simulink model "test_1_cs"  (R2020a)
settings: Solver=ode5  StartTime=0.0  StopTime=150  FixedStep=1/1000  RelTol=1e-3
PreLoadFcn:
  | mbxruntime.callbacks.PreLoadFcn(bdroot);
PostLoadFcn:
  | mbxruntime.callbacks.PostLoadFcn(bdroot);
InitFcn:
  | mbxruntime.callbacks.InitFcn(bdroot);
StartFcn:
  | mbxruntime.callbacks.StartFcn(bdroot);
StopFcn:
  | mbxruntime.callbacks.StopFcn(bdroot);
model workspace (MAT data in the model file):
  mbox_table : object (value not decoded)
  model_closed = 0
  sim_status = 0
undefined symbols (not defined in the file or in its folder): aubr, c_factor, cf, cr, DiscIntNeverNeededParam, global_path_x, global_path_y, KD_PID_distance, KD_PID_speed, KI_PID_distance, KI_PID_speed, KP_PID_distance, KP_PID_speed, la, lb, LQR_K1, LQR_K2, LQR_K3, LQR_K4, m, rack_displacement, right_wheel_ground, tablebr, vubr, vx_break_point
libraries: PreScanSimulinkLibrary x48, simulink_extras x5, simulink x3, Solver_SF x1
(part 8 of 12)

== system test_1_cs/Audi_A8_Sedan_1/control module/control main/longitudinal control double PID ==
  s_err[m] : Inport
  speed_desire[m/s] : Inport  Port=2
  accelerate desire[m/s^2] : Inport  Port=3
  host_speed[m/s] : Inport  Port=4
  host_s_dot[m/s] : Inport  Port=5
  KP_PID_distance : Inport  Port=6
  KI_PID_distance : Inport  Port=7
  KD_PID_distance : Inport  Port=8
  KP_PID_speed : Inport  Port=9
  KI_PID_speed : Inport  Port=10
  KD_PID_speed : Inport  Port=11
  2-D Lookup Table : Lookup_n-D  BreakpointsForDimension1=vubr  BreakpointsForDimension2=aubr  Table=tablebr  InternalRulePriority=Speed  RndMeth=Simplest  InputSameDT=on
  Add : Sum  Inputs=++-
  Add1 : Sum
  Bus Creator : BusCreator  Inputs=9
  Constant : Constant  Value=50
  Constant1 : Constant  Value=50
  Discrete Filter : DiscreteFilter
  MATLAB Function1 : MATLAB Function  TreatAsAtomicUnit=on
  Saturation : Saturate  UpperLimit=45  LowerLimit=-45
  Saturation1 : Saturate  UpperLimit=5  LowerLimit=-8
  Scope1 : Scope
  Scope2 : Scope
  distance pid : simulink/Continuous/PID Controller  Controller=PID  Form=Parallel  TimeDomain=Continuous-time  UseExternalTs=off  SampleTime=-1  IntegratorMethod=Forward Euler  FilterMethod=Forward Euler  ControllerParametersSource=external  P=1  I=1  D=0  UseFilter=on  N=100  TunerSelectOption=Transfer Function Based (PID Tuner App)  InitialConditionSource=internal  InitialConditionForIntegrator=0  InitialConditionForFilter=0  DifferentiatorICPrevScaledInput=0  ExternalReset=none  TrackingMode=off  Kt=1  LimitOutput=off  UpperSaturationLimit=inf  LowerSaturationLimit=-inf  LinearizeAsGain=on  AntiWindupMode=none  Kb=1  POutMin=[]  POutMax=[]  IOutMin=[]  IOutMax=[]  DOutMin=[]  DOutMax=[]  NOutMin=[]  NOutMax=[]  SumOutMin=[]  SumOutMax=[]  SaturationOutMin=[]  SaturationOutMax=[]  PParamMin=[]  PParamMax=[]  IParamMin=[]  IParamMax=[]  DParamMin=[]  DParamMax=[]  NParamMin=[]  NParamMax=[]  KbParamMin=[]  KbParamMax=[]  KtParamMin=[]  KtParamMax=[]  KbOutMin=[]  KbOutMax=[]  KtOutMin=[]  KtOutMax=[]  IntegratorOutMin=[]  IntegratorOutMax=[]  FilterOutMin=[]  FilterOutMax=[]  SumI1OutMin=[]  SumI1OutMax=[]  SumI2OutMin=[]  SumI2OutMax=[]  SumI3OutMin=[]  SumI3OutMax=[]  SumI4OutMin=[]  SumI4OutMax=[]  SumDOutMin=[]  SumDOutMax=[]  DifferentiatorOutMin=[]  DifferentiatorOutMax=[]  FilterDiffOutCoefMin=[]  FilterDiffOutCoefMax=[]  ReciprocalOutMin=[]  ReciprocalOutMax=[]  SumDenOutMin=[]  SumDenOutMax=[]  SumNumOutMin=[]  SumNumOutMax=[]  DivideOutMin=[]  DivideOutMax=[]  UdiffTsProdOutMin=[]  UdiffTsProdOutMax=[]  NTsProdOutMin=[]  NTsProdOutMax=[]  UintegralTsProdOutMin=[]  UintegralTsProdOutMax=[]  UngainTsProdOutMin=[]  UngainTsProdOutMax=[]  IntegratorContinuousStateAttributes=''  IntegratorStateMustResolveToSignalObject=off  IntegratorRTWStateStorageClass=Auto  FilterContinuousStateAttributes=''  FilterStateMustResolveToSignalObject=off  FilterRTWStateStorageClass=Auto  ParallelPVariant=ExternalParameters  IdealPVariant=Disabled  IVariant=ExternalParameters  DVariant=ExternalParameters  IntegratorVariant=Continuous  SatVariant=Disabled  AWVariant=Passthrough  PCopyVariant=Disabled  TRVariant=Disabled  FdbkBlocksVariant=Forward  IdealPFdbkVariant=Disabled  SatFdbkVariant=Disabled  DerivativeFilterVariant=ContFilter  NVariant=ExternalParameters  NCopyVariant=Disabled  FilterICVariant=InternalICsFilter  IntegratorICVariant=InternalICs  ExternalResetVariant=Disabled  TRSumVariant=Passthrough  SumFdbkVariant=Disabled  SumVariant=Sum_PID  TsampFilterVariant=InternalTs  TsampNgainVariant=Passthrough  TsampIntegralVariant=Passthrough
  speed pid : simulink/Continuous/PID Controller  Controller=PID  Form=Parallel  TimeDomain=Continuous-time  UseExternalTs=off  SampleTime=-1  IntegratorMethod=Forward Euler  FilterMethod=Forward Euler  ControllerParametersSource=external  P=1  I=1  D=0  UseFilter=on  N=100  TunerSelectOption=Transfer Function Based (PID Tuner App)  InitialConditionSource=internal  InitialConditionForIntegrator=0  InitialConditionForFilter=0  DifferentiatorICPrevScaledInput=0  ExternalReset=none  TrackingMode=off  Kt=1  LimitOutput=off  UpperSaturationLimit=inf  LowerSaturationLimit=-inf  LinearizeAsGain=on  AntiWindupMode=none  Kb=1  POutMin=[]  POutMax=[]  IOutMin=[]  IOutMax=[]  DOutMin=[]  DOutMax=[]  NOutMin=[]  NOutMax=[]  SumOutMin=[]  SumOutMax=[]  SaturationOutMin=[]  SaturationOutMax=[]  PParamMin=[]  PParamMax=[]  IParamMin=[]  IParamMax=[]  DParamMin=[]  DParamMax=[]  NParamMin=[]  NParamMax=[]  KbParamMin=[]  KbParamMax=[]  KtParamMin=[]  KtParamMax=[]  KbOutMin=[]  KbOutMax=[]  KtOutMin=[]  KtOutMax=[]  IntegratorOutMin=[]  IntegratorOutMax=[]  FilterOutMin=[]  FilterOutMax=[]  SumI1OutMin=[]  SumI1OutMax=[]  SumI2OutMin=[]  SumI2OutMax=[]  SumI3OutMin=[]  SumI3OutMax=[]  SumI4OutMin=[]  SumI4OutMax=[]  SumDOutMin=[]  SumDOutMax=[]  DifferentiatorOutMin=[]  DifferentiatorOutMax=[]  FilterDiffOutCoefMin=[]  FilterDiffOutCoefMax=[]  ReciprocalOutMin=[]  ReciprocalOutMax=[]  SumDenOutMin=[]  SumDenOutMax=[]  SumNumOutMin=[]  SumNumOutMax=[]  DivideOutMin=[]  DivideOutMax=[]  UdiffTsProdOutMin=[]  UdiffTsProdOutMax=[]  NTsProdOutMin=[]  NTsProdOutMax=[]  UintegralTsProdOutMin=[]  UintegralTsProdOutMax=[]  UngainTsProdOutMin=[]  UngainTsProdOutMax=[]  IntegratorContinuousStateAttributes=''  IntegratorStateMustResolveToSignalObject=off  IntegratorRTWStateStorageClass=Auto  FilterContinuousStateAttributes=''  FilterStateMustResolveToSignalObject=off  FilterRTWStateStorageClass=Auto  ParallelPVariant=ExternalParameters  IdealPVariant=Disabled  IVariant=ExternalParameters  DVariant=ExternalParameters  IntegratorVariant=Continuous  SatVariant=Disabled  AWVariant=Passthrough  PCopyVariant=Disabled  TRVariant=Disabled  FdbkBlocksVariant=Forward  IdealPFdbkVariant=Disabled  SatFdbkVariant=Disabled  DerivativeFilterVariant=ContFilter  NVariant=ExternalParameters  NCopyVariant=Disabled  FilterICVariant=InternalICsFilter  IntegratorICVariant=InternalICs  ExternalResetVariant=Disabled  TRSumVariant=Passthrough  SumFdbkVariant=Disabled  SumVariant=Sum_PID  TsampFilterVariant=InternalTs  TsampNgainVariant=Passthrough  TsampIntegralVariant=Passthrough
  throttle : Outport
  brake : Outport  Port=2
  longitudinal_debug : Outport  Port=3
  wires:
  2-D Lookup Table/1 -> Scope2/1, MATLAB Function1/1(u)
  s_err[m]/1 -> [s_err]
  speed_desire[m/s]/1 -> [speed_desire]
  accelerate desire[m/s^2]/1 -> [accelerate_desire]
  KP_PID_distance/1 -> [KP_PID_distance]
  KI_PID_distance/1 -> [KI_PID_distance]
  KD_PID_distance/1 -> [KD_PID_distance]
  KP_PID_speed/1 -> [KP_PID_speed]
  KI_PID_speed/1 -> [KI_PID_speed]
  KD_PID_speed/1 -> [KD_PID_speed]
  Constant/1 -> distance pid/5
  [s_err] -> Discrete Filter/1
  [KP_PID_distance] -> distance pid/2
  [KI_PID_distance] -> distance pid/3
  [KD_PID_distance] -> distance pid/4
  Constant1/1 -> speed pid/5
  [KP_PID_speed] -> speed pid/2
  [KI_PID_speed] -> speed pid/3
  [KD_PID_speed] -> speed pid/4
  host_speed[m/s]/1 -> [host_speed]
  distance pid/1 -> Add/1
  [speed_desire] -> Add/2
  Add/1 -> Saturation/1
  Saturation/1 -> speed pid/1
  speed pid/1 -> Add1/1
  [accelerate_desire] -> Add1/2
  Add1/1 -> Saturation1/1
  Saturation1/1 -> Scope1/1, 2-D Lookup Table/2
  host_s_dot[m/s]/1 -> [host_s_dot]
  [host_s_dot] -> Add/3
  [host_speed] -> 2-D Lookup Table/1
  Discrete Filter/1 -> distance pid/1
  MATLAB Function1/1(throttle) -> throttle/1
  MATLAB Function1/2(brake) -> brake/1
  [KP_PID_distance] -> Bus Creator/1  "KP_PID_distance"
  [KI_PID_distance] -> Bus Creator/2  "KI_PID_distance"
  [KD_PID_distance] -> Bus Creator/3  "KD_PID_distance"
  [KP_PID_speed] -> Bus Creator/4  "KP_PID_speed"
  [KI_PID_speed] -> Bus Creator/5  "KI_PID_speed"
  [KD_PID_speed] -> Bus Creator/6  "KD_PID_speed"
  [host_speed] -> Bus Creator/7  "host_speed"
  [s_err] -> Bus Creator/8  "s_err"
  [host_s_dot] -> Bus Creator/9  "host_s_dot"
  Bus Creator/1 -> longitudinal_debug/1

== system test_1_cs/Audi_A8_Sedan_1/control module/control main/understeer compensate ==
  LQR_angle : Inport
  lateral err : Inport  Port=2
  Add : Sum  Inputs=+-
  Gain : Gain  Gain=0.01
  Integrator : Integrator
  Manual Switch : ManualSwitch
  LQR_final_angle : Outport
  wires:
  Integrator/1 -> Gain/1
  Add/1 -> Manual Switch/2
  lateral err/1 -> Integrator/1
  Manual Switch/1 -> LQR_final_angle/1
  LQR_angle/1 -> Add/1, Manual Switch/1
  Gain/1 -> Add/2

== system test_1_cs/Audi_A8_Sedan_1/control module1/control main/chassic steering system ==
  LQR_final_angle : Inport
  Constant : Constant  Value=la
  Constant1 : Constant  Value=lb
  Constant17 : Constant  Value=c_factor
  Divide : Product  Inputs=*/
  Gain3 : Gain  Gain=180/pi
  Gain4 : Gain  Gain=360
  MATLAB Function : MATLAB Function  TreatAsAtomicUnit=on
  Saturation : Saturate  UpperLimit=70  LowerLimit=-70
  Saturation1 : Saturate  UpperLimit=1.2217  LowerLimit=-1.2217
  transfer right wheel angle to rack displancement : Lookup_n-D  NumberOfTableDimensions=1  BreakpointsForDimension1=right_wheel_ground  Table=rack_displacement  InternalRulePriority=Speed  RndMeth=Simplest  InputSameDT=on
  lat_steer_sw[deg] : Outport
  wires:
  transfer right wheel angle to rack displancement/1 -> Divide/1
  Constant17/1 -> Divide/2
  Gain4/1 -> lat_steer_sw[deg]/1
  Divide/1 -> Gain4/1
  Saturation/1 -> transfer right wheel angle to rack displancement/1
  Constant/1 -> MATLAB Function/2(la)
  Gain3/1 -> Saturation/1
  Constant1/1 -> MATLAB Function/3(lb)
  LQR_final_angle/1 -> Saturation1/1
  Saturation1/1 -> MATLAB Function/1(u)
  MATLAB Function/1(right_steer) -> Gain3/1

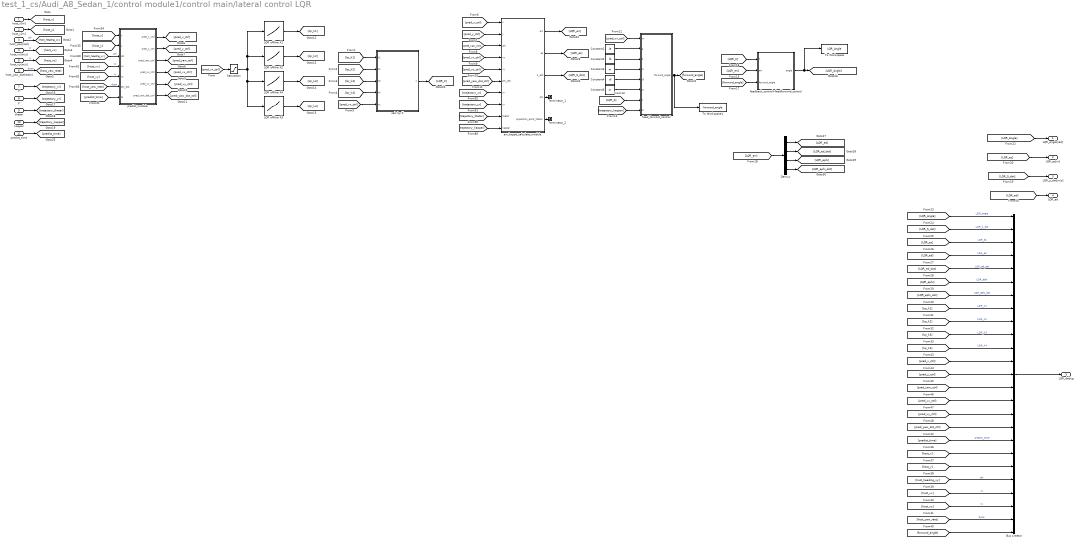
== system test_1_cs/Audi_A8_Sedan_1/control module1/control main/lateral control LQR ==
  host_x[m] : Inport
  host_y[m] : Inport  Port=2
  host_yaw[rad] : Inport  Port=3
  host_vx[m/s] : Inport  Port=4
  host_vy[m/s] : Inport  Port=5
  host_yaw_dot[rad/s] : Inport  Port=6
  xr : Inport  Port=7
  yr : Inport  Port=8
  thetar : Inport  Port=9
  kappar : Inport  Port=10
  predict_time : Inport  Port=11
  Bus Creator : BusCreator  Inputs=25
  Constant1 : Constant  Value=la
  Constant2 : Constant  Value=lb
  Constant3 : Constant  Value=m
  Constant4 : Constant  Value=cf
  Constant5 : Constant  Value=cr
  Demux : Demux
  LQR offline K1 : Lookup_n-D  NumberOfTableDimensions=1  BreakpointsForDimension1=vx_break_point  Table=LQR_K1  InternalRulePriority=Speed  RndMeth=Simplest  InputSameDT=on
  LQR offline K2 : Lookup_n-D  NumberOfTableDimensions=1  BreakpointsForDimension1=vx_break_point  Table=LQR_K2  InternalRulePriority=Speed  RndMeth=Simplest  InputSameDT=on
  LQR offline K3 : Lookup_n-D  NumberOfTableDimensions=1  BreakpointsForDimension1=vx_break_point  Table=LQR_K3  InternalRulePriority=Speed  RndMeth=Simplest  InputSameDT=on
  LQR offline K4 : Lookup_n-D  NumberOfTableDimensions=1  BreakpointsForDimension1=vx_break_point  Table=LQR_K4  InternalRulePriority=Speed  RndMeth=Simplest  InputSameDT=on
  Saturation : Saturate  UpperLimit=50  LowerLimit=0
  Terminator_1 : Terminator
  Terminator_2 : Terminator
  To Workspace : ToWorkspace  VariableName=LQR_Angle  SaveFormat=Timeseries  SampleTime=-1
  To Workspace1 : ToWorkspace  VariableName=forward_angle  SaveFormat=Timeseries  SampleTime=-1
  calc lqr K : MATLAB Function  TreatAsAtomicUnit=on
  err_kappa_calculate_module : MATLAB Function  TreatAsAtomicUnit=on
  feed_forword_control : MATLAB Function  TreatAsAtomicUnit=on
  feedback_control+feedforword_control : MATLAB Function  TreatAsAtomicUnit=on
  predict_module : MATLAB Function  TreatAsAtomicUnit=on
  LQR_angle[rad] : Outport  VectorParamsAs1DForOutWhenUnconnected=off
  LQR_es[m] : Outport  Port=2  VectorParamsAs1DForOutWhenUnconnected=off
  LQR_s_dot[m/s] : Outport  Port=3  VectorParamsAs1DForOutWhenUnconnected=off
  LQR_ed : Outport  Port=4  VectorParamsAs1DForOutWhenUnconnected=off
  LQR_debug : Outport  Port=5  VectorParamsAs1DForOutWhenUnconnected=off
  wires:
  [host_vy] -> predict_module/5(vy)  "vy"
  [host_x] -> predict_module/1(x)
  [host_yaw_rate] -> predict_module/6(phi_dot)  "dyaw"
  [host_vx] -> predict_module/4(vx)  "vx"
  [host_y] -> predict_module/2(y)
  [host_heading_xy] -> predict_module/3(phi)  "phi"
  [predict_time] -> predict_module/7(ts)
  host_x[m]/1 -> [host_x]
  host_y[m]/1 -> [host_y]
  host_yaw[rad]/1 -> [host_heading_xy]  "phi"
  host_vx[m/s]/1 -> [host_vx]  "vx"
  host_vy[m/s]/1 -> [host_vy]  "vy"
  host_yaw_dot[rad/s]/1 -> [host_yaw_rate]  "dyaw"
  predict_module/1(pred_x_ctrl) -> [pred_x_ctrl]
  predict_module/2(pred_y_ctrl) -> [pred_y_ctrl]
  predict_module/3(pred_yaw_ctrl) -> [pred_yaw_ctrl]
  predict_module/4(pred_vx_ctrl) -> [pred_vx_ctrl]
  predict_module/5(pred_vy_ctrl) -> [pred_vy_ctrl]
  predict_module/6(pred_yaw_dot_ctrl) -> [pred_yaw_dot_ctrl]
  [pred_vx_ctrl] -> Saturation/1
  LQR offline K1/1 -> [lqr_k1]
  LQR offline K2/1 -> [lqr_k2]
  LQR offline K4/1 -> [lqr_k3]
  LQR offline K3/1 -> [lqr_k4]
  [pred_vx_ctrl] -> calc lqr K/5(vx)
  [lqr_k4] -> calc lqr K/4(k4)
  [lqr_k3] -> calc lqr K/3(k3)
  [lqr_k2] -> calc lqr K/2(k2)
  [lqr_k1] -> calc lqr K/1(k1)
  [pred_x_ctrl] -> err_kappa_calculate_module/1(x)
  [pred_y_ctrl] -> err_kappa_calculate_module/2(y)
  [pred_yaw_ctrl] -> err_kappa_calculate_module/3("phi ")
  [pred_vx_ctrl] -> err_kappa_calculate_module/4(vx)
  [pred_vy_ctrl] -> err_kappa_calculate_module/5(vy)
  [pred_yaw_dot_ctrl] -> err_kappa_calculate_module/6(phi_dot)
  xr/1 -> [trajectory_xr]
  yr/1 -> [trajectory_yr]
  thetar/1 -> [trajectory_thetar]
  kappar/1 -> [trajectory_kappar]
  [trajectory_xr] -> err_kappa_calculate_module/7(xr)
  [trajectory_yr] -> err_kappa_calculate_module/8(yr)
  [trajectory_kappar] -> err_kappa_calculate_module/10(kappar)
  [trajectory_thetar] -> err_kappa_calculate_module/9(thetar)
  [pred_vx_ctrl] -> feed_forword_control/1(vx)
  Constant1/1 -> feed_forword_control/2(a)
  Constant2/1 -> feed_forword_control/3(b)
  Constant3/1 -> feed_forword_control/4(m)
  Constant4/1 -> feed_forword_control/5(cf)
  Constant5/1 -> feed_forword_control/6(cr)
  calc lqr K/1(k) -> [LQR_K]
  [LQR_K] -> feed_forword_control/7(k)
  [trajectory_kappar] -> feed_forword_control/8(kr)
  feed_forword_control/1(forword_angle) -> To Workspace1/1, [forword_angle]
  err_kappa_calculate_module/1(err) -> [LQR_err]
  [LQR_err] -> feedback_control+feedforword_control/2(err)
  [LQR_K] -> feedback_control+feedforword_control/1(k)
  [forword_angle] -> feedback_control+feedforword_control/3(forword_angle)
  [LQR_err] -> Demux/1
  err_kappa_calculate_module/2(es) -> [LQR_es]
  err_kappa_calculate_module/3(s_dot) -> [LQR_S_dot]
  [LQR_S_dot] -> LQR_s_dot[m/s]/1
  [LQR_es] -> LQR_es[m]/1
  Saturation/1 -> LQR offline K3/1, LQR offline K4/1, LQR offline K2/1, LQR offline K1/1
  predict_time/1 -> [predict_time]
  Bus Creator/1 -> LQR_debug/1
  feedback_control+feedforword_control/1(angle) -> To Workspace/1, [LQR_Angle]
  [LQR_Angle] -> LQR_angle[rad]/1
  [LQR_Angle] -> Bus Creator/1  "LQR_angle"
  [LQR_S_dot] -> Bus Creator/2  "LQR_s_dot"
  [LQR_es] -> Bus Creator/3  "LQR_es"
  Demux/1 -> [LQR_ed]
  Demux/2 -> [LQR_ed_dot]
  Demux/3 -> [LQR_ephi]
  Demux/4 -> [LQR_ephi_dot]
  [LQR_ed] -> Bus Creator/4  "LQR_ed"
  [LQR_ed_dot] -> Bus Creator/5  "LQR_ed_dot"
  [LQR_ephi] -> Bus Creator/6  "LQR_ephi"
  [LQR_ephi_dot] -> Bus Creator/7  "LQR_ephi_dot"
  [lqr_k1] -> Bus Creator/8  "LQR_K1"
  [lqr_k2] -> Bus Creator/9  "LQR_K2"
  [lqr_k3] -> Bus Creator/10  "LQR_K3"
  [lqr_k4] -> Bus Creator/11  "LQR_K4"
  [pred_x_ctrl] -> Bus Creator/12
  [pred_y_ctrl] -> Bus Creator/13
  [pred_yaw_ctrl] -> Bus Creator/14
  [pred_vx_ctrl] -> Bus Creator/15
  [pred_vy_ctrl] -> Bus Creator/16
  [pred_yaw_dot_ctrl] -> Bus Creator/17
  [predict_time] -> Bus Creator/18  "predict_time"
  [host_x] -> Bus Creator/19
  [host_y] -> Bus Creator/20
  [host_heading_xy] -> Bus Creator/21  "phi"
  [host_vx] -> Bus Creator/22  "vx"
  [host_vy] -> Bus Creator/23  "vy"
  [host_yaw_rate] -> Bus Creator/24  "dyaw"
  [forword_angle] -> Bus Creator/25
  [LQR_ed] -> LQR_ed/1
  err_kappa_calculate_module/4(phi) -> Terminator_1/1
  err_kappa_calculate_module/5(projection_point_thetar) -> Terminator_2/1

== system test_1_cs/Audi_A8_Sedan_1/control module1/control main/longitudinal control double PID ==
  s_err[m] : Inport
  speed_desire[m/s] : Inport  Port=2
  accelerate desire[m/s^2] : Inport  Port=3
  host_speed[m/s] : Inport  Port=4
  host_s_dot[m/s] : Inport  Port=5
  KP_PID_distance : Inport  Port=6
  KI_PID_distance : Inport  Port=7
  KD_PID_distance : Inport  Port=8
  KP_PID_speed : Inport  Port=9
  KI_PID_speed : Inport  Port=10
  KD_PID_speed : Inport  Port=11
  2-D Lookup Table : Lookup_n-D  BreakpointsForDimension1=vubr  BreakpointsForDimension2=aubr  Table=tablebr  InternalRulePriority=Speed  RndMeth=Simplest  InputSameDT=on
  Add : Sum  Inputs=++-
  Add1 : Sum
  Bus Creator : BusCreator  Inputs=9
  Discrete Filter : DiscreteFilter
  MATLAB Function1 : MATLAB Function  TreatAsAtomicUnit=on
  Saturation : Saturate  UpperLimit=45  LowerLimit=-45
  Saturation1 : Saturate  UpperLimit=5  LowerLimit=-8
  discrete pid distance : Subsystem
  discrete pid speed : Subsystem
  throttle : Outport
  brake : Outport  Port=2
  longitudinal_debug : Outport  Port=3
  wires:
  2-D Lookup Table/1 -> MATLAB Function1/1(u)
  s_err[m]/1 -> [s_err]
  speed_desire[m/s]/1 -> [speed_desire]
  accelerate desire[m/s^2]/1 -> [accelerate_desire]
  KP_PID_distance/1 -> [KP_PID_distance]
  KI_PID_distance/1 -> [KI_PID_distance]
  KD_PID_distance/1 -> [KD_PID_distance]
  KP_PID_speed/1 -> [KP_PID_speed]
  KI_PID_speed/1 -> [KI_PID_speed]
  KD_PID_speed/1 -> [KD_PID_speed]
  [s_err] -> Discrete Filter/1
  host_speed[m/s]/1 -> [host_speed]
  [speed_desire] -> Add/2
  Add/1 -> Saturation/1
  Saturation/1 -> discrete pid speed/1(err)
  discrete pid speed/1(pid_out) -> Add1/1
  [accelerate_desire] -> Add1/2
  Add1/1 -> Saturation1/1
  Saturation1/1 -> 2-D Lookup Table/2
  host_s_dot[m/s]/1 -> [host_s_dot]
  [host_s_dot] -> Add/3
  [host_speed] -> 2-D Lookup Table/1
  MATLAB Function1/1(throttle) -> throttle/1
  MATLAB Function1/2(brake) -> brake/1
  [KP_PID_distance] -> Bus Creator/1  "KP_PID_distance"
  [KI_PID_distance] -> Bus Creator/2  "KI_PID_distance"
  [KD_PID_distance] -> Bus Creator/3  "KD_PID_distance"
  [KP_PID_speed] -> Bus Creator/4  "KP_PID_speed"
  [KI_PID_speed] -> Bus Creator/5  "KI_PID_speed"
  [KD_PID_speed] -> Bus Creator/6  "KD_PID_speed"
  [host_speed] -> Bus Creator/7  "host_speed"
  [s_err] -> Bus Creator/8  "s_err"
  [host_s_dot] -> Bus Creator/9  "host_s_dot"
  Bus Creator/1 -> longitudinal_debug/1
  Discrete Filter/1 -> discrete pid distance/1(err)
  [KP_PID_distance] -> discrete pid distance/2(kp)
  [KI_PID_distance] -> discrete pid distance/3(ki)
  [KD_PID_distance] -> discrete pid distance/4(kd)
  [KP_PID_speed] -> discrete pid speed/2(kp)
  [KI_PID_speed] -> discrete pid speed/3(ki)
  [KD_PID_speed] -> discrete pid speed/4(kd)
  discrete pid distance/1(pid_out) -> Add/1

== system test_1_cs/Audi_A8_Sedan_1/control module1/control main/understeer compensate ==
  LQR_angle : Inport
  lateral err : Inport  Port=2
  Add : Sum  Inputs=+-
  Gain : Gain  Gain=0.01
  Manual Switch : ManualSwitch
  LQR_final_angle : Outport
  wires:
  lateral err/1 -> Gain/1
  Add/1 -> Manual Switch/2
  Manual Switch/1 -> LQR_final_angle/1
  LQR_angle/1 -> Add/1, Manual Switch/1
  Gain/1 -> Add/2

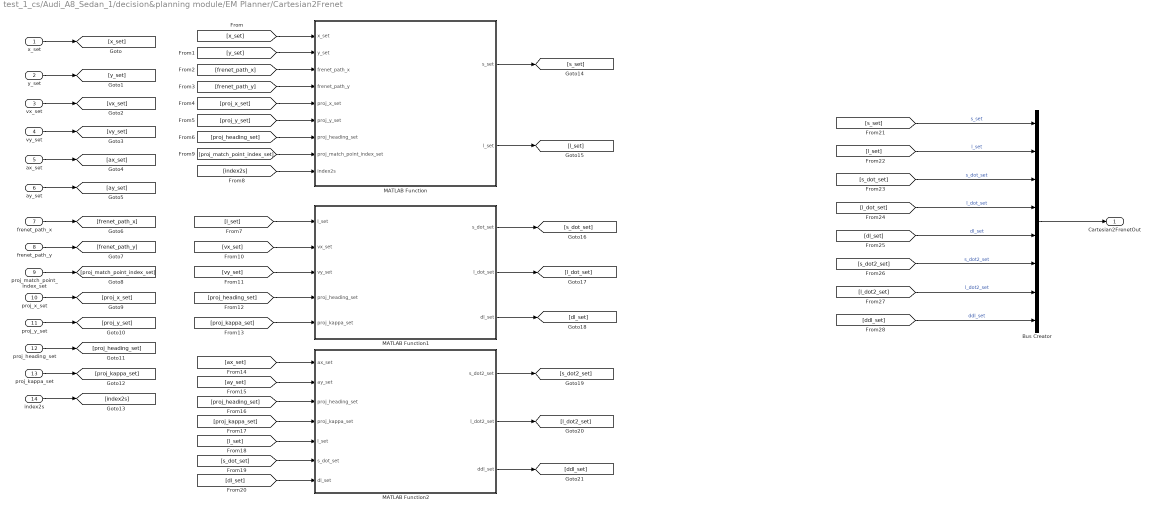
== system test_1_cs/Audi_A8_Sedan_1/decision&planning module/EM Planner/Cartesian2Frenet ==
  x_set : Inport
  y_set : Inport  Port=2
  vx_set : Inport  Port=3
  vy_set : Inport  Port=4
  ax_set : Inport  Port=5
  ay_set : Inport  Port=6
  frenet_path_x : Inport  Port=7
  frenet_path_y : Inport  Port=8
  proj_match_point_index_set : Inport  Port=9
  proj_x_set : Inport  Port=10
  proj_y_set : Inport  Port=11
  proj_heading_set : Inport  Port=12
  proj_kappa_set : Inport  Port=13
  index2s : Inport  Port=14
  Bus Creator : BusCreator  Inputs=8
  MATLAB Function : MATLAB Function  TreatAsAtomicUnit=on
  MATLAB Function1 : MATLAB Function  TreatAsAtomicUnit=on
  MATLAB Function2 : MATLAB Function  TreatAsAtomicUnit=on
  Cartesian2FrenetOut : Outport
  wires:
  x_set/1 -> [x_set]
  y_set/1 -> [y_set]
  vx_set/1 -> [vx_set]
  vy_set/1 -> [vy_set]
  ax_set/1 -> [ax_set]
  ay_set/1 -> [ay_set]
  frenet_path_x/1 -> [frenet_path_x]
  frenet_path_y/1 -> [frenet_path_y]
  proj_match_point_index_set/1 -> [proj_match_point_index_set]
  proj_x_set/1 -> [proj_x_set]
  proj_y_set/1 -> [proj_y_set]
  proj_heading_set/1 -> [proj_heading_set]
  proj_kappa_set/1 -> [proj_kappa_set]
  index2s/1 -> [index2s]
  [x_set] -> MATLAB Function/1(x_set)
  [y_set] -> MATLAB Function/2(y_set)
  [frenet_path_x] -> MATLAB Function/3(frenet_path_x)
  [frenet_path_y] -> MATLAB Function/4(frenet_path_y)
  [proj_x_set] -> MATLAB Function/5(proj_x_set)
  [proj_match_point_index_set] -> MATLAB Function/8(proj_match_point_index_set)
  [proj_y_set] -> MATLAB Function/6(proj_y_set)
  [proj_heading_set] -> MATLAB Function/7(proj_heading_set)
  [index2s] -> MATLAB Function/9(index2s)
  MATLAB Function/1(s_set) -> [s_set]
  MATLAB Function/2(l_set) -> [l_set]
  [l_set] -> MATLAB Function1/1(l_set)
  [vx_set] -> MATLAB Function1/2(vx_set)
  [vy_set] -> MATLAB Function1/3(vy_set)
  [proj_heading_set] -> MATLAB Function1/4(proj_heading_set)
  [proj_kappa_set] -> MATLAB Function1/5(proj_kappa_set)
  [ax_set] -> MATLAB Function2/1(ax_set)
  [ay_set] -> MATLAB Function2/2(ay_set)
  [proj_heading_set] -> MATLAB Function2/3(proj_heading_set)
  [proj_kappa_set] -> MATLAB Function2/4(proj_kappa_set)
  [l_set] -> MATLAB Function2/5(l_set)
  MATLAB Function1/1(s_dot_set) -> [s_dot_set]
  MATLAB Function1/2(l_dot_set) -> [l_dot_set]
  MATLAB Function1/3(dl_set) -> [dl_set]
  [s_dot_set] -> MATLAB Function2/6(s_dot_set)
  [dl_set] -> MATLAB Function2/7(dl_set)
  MATLAB Function2/1(s_dot2_set) -> [s_dot2_set]
  MATLAB Function2/2(l_dot2_set) -> [l_dot2_set]
  MATLAB Function2/3(ddl_set) -> [ddl_set]
  [s_set] -> Bus Creator/1  "s_set"
  [l_set] -> Bus Creator/2  "l_set"
  [s_dot_set] -> Bus Creator/3  "s_dot_set"
  [l_dot_set] -> Bus Creator/4  "l_dot_set"
  [dl_set] -> Bus Creator/5  "dl_set"
  [s_dot2_set] -> Bus Creator/6  "s_dot2_set"
  [l_dot2_set] -> Bus Creator/7  "l_dot2_set"
  [ddl_set] -> Bus Creator/8  "ddl_set"
  Bus Creator/1 -> Cartesian2FrenetOut/1

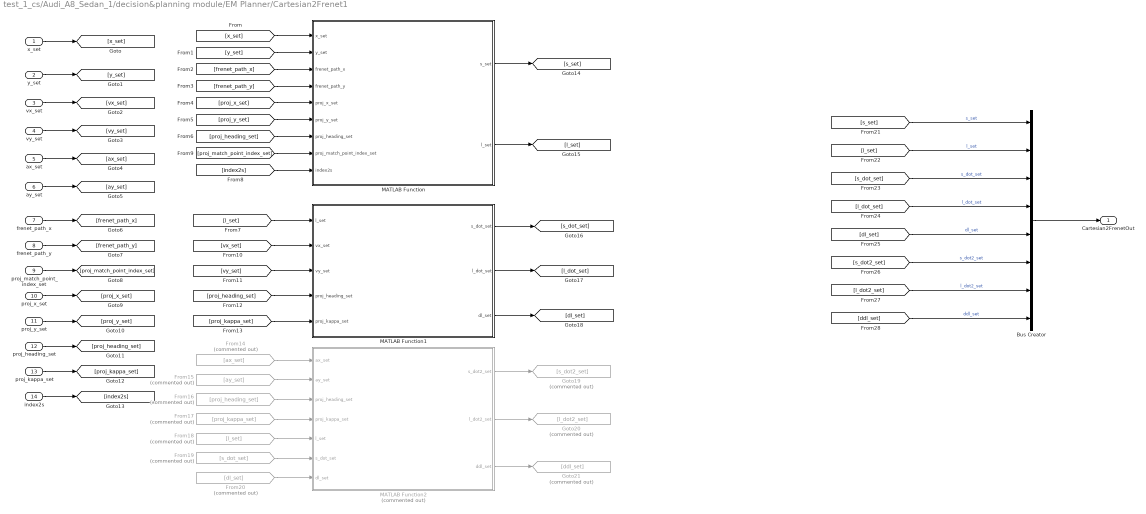
== system test_1_cs/Audi_A8_Sedan_1/decision&planning module/EM Planner/Cartesian2Frenet1 ==
  x_set : Inport
  y_set : Inport  Port=2
  vx_set : Inport  Port=3
  vy_set : Inport  Port=4
  ax_set : Inport  Port=5
  ay_set : Inport  Port=6
  frenet_path_x : Inport  Port=7
  frenet_path_y : Inport  Port=8
  proj_match_point_index_set : Inport  Port=9
  proj_x_set : Inport  Port=10
  proj_y_set : Inport  Port=11
  proj_heading_set : Inport  Port=12
  proj_kappa_set : Inport  Port=13
  index2s : Inport  Port=14
  Bus Creator : BusCreator  Inputs=8
  From14 : From  Commented=on  GotoTag=ax_set
  From15 : From  Commented=on  GotoTag=ay_set
  From16 : From  Commented=on  GotoTag=proj_heading_set
  From17 : From  Commented=on  GotoTag=proj_kappa_set
  From18 : From  Commented=on  GotoTag=l_set
  From19 : From  Commented=on  GotoTag=s_dot_set
  From20 : From  Commented=on  GotoTag=dl_set
  Goto19 : Goto  Commented=on  GotoTag=s_dot2_set
  Goto20 : Goto  Commented=on  GotoTag=l_dot2_set
  Goto21 : Goto  Commented=on  GotoTag=ddl_set
  MATLAB Function : MATLAB Function  TreatAsAtomicUnit=on
  MATLAB Function1 : MATLAB Function  TreatAsAtomicUnit=on
  MATLAB Function2 : MATLAB Function  Commented=on  TreatAsAtomicUnit=on
  Cartesian2FrenetOut : Outport
  wires:
  Bus Creator/1 -> Cartesian2FrenetOut/1
  [ddl_set] -> Bus Creator/8  "ddl_set"
  [l_dot2_set] -> Bus Creator/7  "l_dot2_set"
  [s_dot2_set] -> Bus Creator/6  "s_dot2_set"
  [dl_set] -> Bus Creator/5  "dl_set"
  [l_dot_set] -> Bus Creator/4  "l_dot_set"
  [s_dot_set] -> Bus Creator/3  "s_dot_set"
  [l_set] -> Bus Creator/2  "l_set"
  [s_set] -> Bus Creator/1  "s_set"
  MATLAB Function2/3(ddl_set) -> Goto21/1
  MATLAB Function2/2(l_dot2_set) -> Goto20/1
  MATLAB Function2/1(s_dot2_set) -> Goto19/1
  From20/1 -> MATLAB Function2/7(dl_set)
  From19/1 -> MATLAB Function2/6(s_dot_set)
  MATLAB Function1/3(dl_set) -> [dl_set]
  MATLAB Function1/2(l_dot_set) -> [l_dot_set]
  MATLAB Function1/1(s_dot_set) -> [s_dot_set]
  From18/1 -> MATLAB Function2/5(l_set)
  From17/1 -> MATLAB Function2/4(proj_kappa_set)
  From16/1 -> MATLAB Function2/3(proj_heading_set)
  From15/1 -> MATLAB Function2/2(ay_set)
  From14/1 -> MATLAB Function2/1(ax_set)
  [proj_kappa_set] -> MATLAB Function1/5(proj_kappa_set)
  [proj_heading_set] -> MATLAB Function1/4(proj_heading_set)
  [vy_set] -> MATLAB Function1/3(vy_set)
  [vx_set] -> MATLAB Function1/2(vx_set)
  [l_set] -> MATLAB Function1/1(l_set)
  MATLAB Function/2(l_set) -> [l_set]
  MATLAB Function/1(s_set) -> [s_set]
  [index2s] -> MATLAB Function/9(index2s)
  [proj_heading_set] -> MATLAB Function/7(proj_heading_set)
  [proj_y_set] -> MATLAB Function/6(proj_y_set)
  [proj_match_point_index_set] -> MATLAB Function/8(proj_match_point_index_set)
  [proj_x_set] -> MATLAB Function/5(proj_x_set)
  [frenet_path_y] -> MATLAB Function/4(frenet_path_y)
  [frenet_path_x] -> MATLAB Function/3(frenet_path_x)
  [y_set] -> MATLAB Function/2(y_set)
  [x_set] -> MATLAB Function/1(x_set)
  index2s/1 -> [index2s]
  proj_kappa_set/1 -> [proj_kappa_set]
  proj_heading_set/1 -> [proj_heading_set]
  proj_y_set/1 -> [proj_y_set]
  proj_x_set/1 -> [proj_x_set]
  proj_match_point_index_set/1 -> [proj_match_point_index_set]
  frenet_path_y/1 -> [frenet_path_y]
  frenet_path_x/1 -> [frenet_path_x]
  ay_set/1 -> [ay_set]
  ax_set/1 -> [ax_set]
  vy_set/1 -> [vy_set]
  vx_set/1 -> [vx_set]
  y_set/1 -> [y_set]
  x_set/1 -> [x_set]

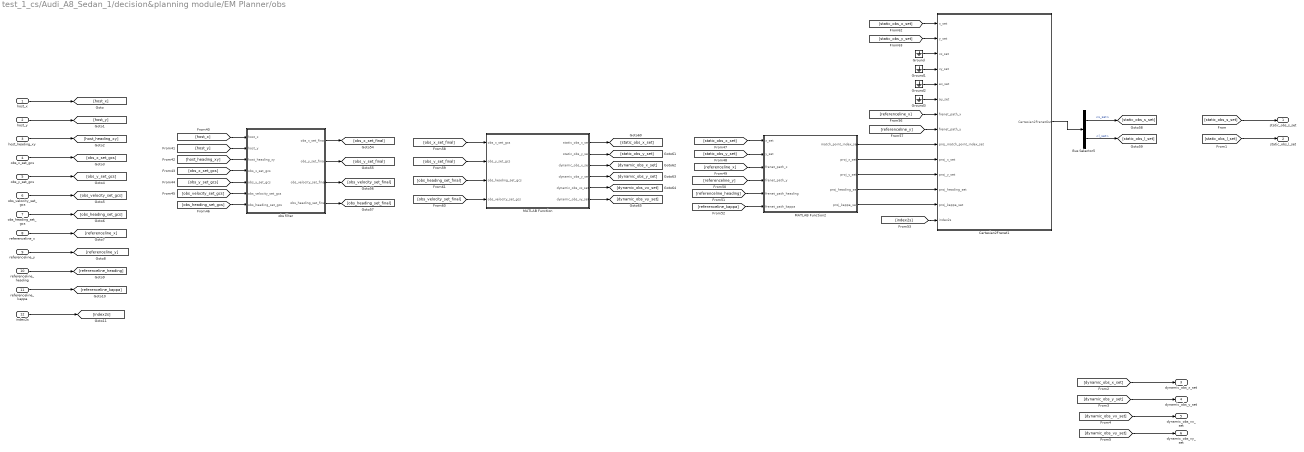
== system test_1_cs/Audi_A8_Sedan_1/decision&planning module/EM Planner/obs ==
  host_x : Inport
  host_y : Inport  Port=2
  host_heading_xy : Inport  Port=3
  obs_x_set_gcs : Inport  Port=4
  obs_y_set_gcs : Inport  Port=5
  obs_velocity_set_gcs : Inport  Port=6
  obs_heading_set_gcs : Inport  Port=7
  referenceline_x : Inport  Port=8
  referenceline_y : Inport  Port=9
  referenceline_heading : Inport  Port=10
  referenceline_kappa : Inport  Port=11
  index2s : Inport  Port=12
  Bus Selector5 : BusSelector  OutputSignals=s_set,l_set
  Cartesian2Frenet1 : Subsystem
  Ground{,1..3} (4 alike) : Ground
  MATLAB Function : MATLAB Function  TreatAsAtomicUnit=on
  MATLAB Function2 : MATLAB Function  TreatAsAtomicUnit=on
  obs filter : MATLAB Function  TreatAsAtomicUnit=on
  static_obs_s_set : Outport
  static_obs_l_set : Outport  Port=2
  dynamic_obs_x_set : Outport  Port=3
  dynamic_obs_y_set : Outport  Port=4
  dynamic_obs_vx_set : Outport  Port=5
  dynamic_obs_vy_set : Outport  Port=6
  wires:
  Ground3/1 -> Cartesian2Frenet1/6(ay_set)
  [obs_x_set_gcs] -> obs filter/4(obs_x_set_gcs)
  [index2s] -> Cartesian2Frenet1/14(index2s)
  [referenceline_y] -> Cartesian2Frenet1/8(frenet_path_y)
  MATLAB Function2/5(proj_kappa_set) -> Cartesian2Frenet1/13(proj_kappa_set)
  MATLAB Function2/4(proj_heading_set) -> Cartesian2Frenet1/12(proj_heading_set)
  [referenceline_x] -> MATLAB Function2/3(frenet_path_x)
  Ground2/1 -> Cartesian2Frenet1/5(ax_set)
  obs filter/1(obs_x_set_final) -> [obs_x_set_final]
  obs filter/4(obs_heading_set_final) -> [obs_heading_set_final]
  [host_heading_xy] -> obs filter/3(host_heading_xy)
  MATLAB Function/5(dynamic_obs_vx_set) -> [dynamic_obs_vx_set]
  [obs_y_set_final] -> MATLAB Function/2(obs_y_set_gcs)
  MATLAB Function/6(dynamic_obs_vy_set) -> [dynamic_obs_vy_set]
  [referenceline_y] -> MATLAB Function2/4(frenet_path_y)
  obs filter/3(obs_velocity_set_final) -> [obs_velocity_set_final]
  MATLAB Function/1(static_obs_x_set) -> [static_obs_x_set]
  [obs_heading_set_gcs] -> obs filter/7(obs_heading_set_gcs)
  [referenceline_kappa] -> MATLAB Function2/6(frenet_path_kappa)
  [static_obs_x_set] -> Cartesian2Frenet1/1(x_set)
  [static_obs_y_set] -> MATLAB Function2/2(y_set)
  [referenceline_x] -> Cartesian2Frenet1/7(frenet_path_x)
  Ground1/1 -> Cartesian2Frenet1/4(vy_set)
  [obs_x_set_final] -> MATLAB Function/1(obs_x_set_gcs)
  [obs_velocity_set_gcs] -> obs filter/6(obs_velocity_set_gcs)
  [host_y] -> obs filter/2(host_y)
  Bus Selector5/2 -> [static_obs_l_set]  "<l_set>"
  [referenceline_heading] -> MATLAB Function2/5(frenet_path_heading)
  obs filter/2(obs_y_set_final) -> [obs_y_set_final]
  Bus Selector5/1 -> [static_obs_s_set]  "<s_set>"
  MATLAB Function/3(dynamic_obs_x_set) -> [dynamic_obs_x_set]
  MATLAB Function2/2(proj_x_set) -> Cartesian2Frenet1/10(proj_x_set)
  Ground/1 -> Cartesian2Frenet1/3(vx_set)
  MATLAB Function2/3(proj_y_set) -> Cartesian2Frenet1/11(proj_y_set)
  MATLAB Function/4(dynamic_obs_y_set) -> [dynamic_obs_y_set]
  MATLAB Function2/1(match_point_index_set) -> Cartesian2Frenet1/9(proj_match_point_index_set)
  [host_x] -> obs filter/1(host_x)
  [obs_y_set_gcs] -> obs filter/5(obs_y_set_gcs)
  Cartesian2Frenet1/1(Cartesian2FrenetOut) -> Bus Selector5/1
  [static_obs_x_set] -> MATLAB Function2/1(x_set)
  MATLAB Function/2(static_obs_y_set) -> [static_obs_y_set]
  [static_obs_y_set] -> Cartesian2Frenet1/2(y_set)
  host_x/1 -> [host_x]
  host_y/1 -> [host_y]
  host_heading_xy/1 -> [host_heading_xy]
  obs_x_set_gcs/1 -> [obs_x_set_gcs]
  obs_y_set_gcs/1 -> [obs_y_set_gcs]
  obs_velocity_set_gcs/1 -> [obs_velocity_set_gcs]
  obs_heading_set_gcs/1 -> [obs_heading_set_gcs]
  referenceline_x/1 -> [referenceline_x]
  referenceline_y/1 -> [referenceline_y]
  referenceline_heading/1 -> [referenceline_heading]
  referenceline_kappa/1 -> [referenceline_kappa]
  index2s/1 -> [index2s]
  [static_obs_s_set] -> static_obs_s_set/1
  [static_obs_l_set] -> static_obs_l_set/1
  [dynamic_obs_vy_set] -> dynamic_obs_vy_set/1
  [dynamic_obs_vx_set] -> dynamic_obs_vx_set/1
  [dynamic_obs_y_set] -> dynamic_obs_y_set/1
  [dynamic_obs_x_set] -> dynamic_obs_x_set/1
  [obs_velocity_set_final] -> MATLAB Function/4(obs_velocity_set_gcs)
  [obs_heading_set_final] -> MATLAB Function/3(obs_heading_set_gcs)

== system test_1_cs/Audi_A8_Sedan_1/decision&planning module/EM Planner/path decision task ==
  static_obs_s_set : Inport
  static_obs_l_set : Inport  Port=2
  plan_start_s : Inport  Port=3
  plan_start_l : Inport  Port=4
  plan_start_dl : Inport  Port=5
  plan_start_ddl : Inport  Port=6
  dp_cost_collision : Inport  Port=7
  dp_cost_dl : Inport  Port=8
  dp_cost_ddl : Inport  Port=9
  dp_cost_dddl : Inport  Port=10
  dp_cost_ref : Inport  Port=11
  dp_row : Inport  Port=12
  dp_col : Inport  Port=13
  dp_sample_s : Inport  Port=14
  dp_sample_l : Inport  Port=15
  increase DP path nodes : MATLAB Function  TreatAsAtomicUnit=on
  path decision with dynamic planning(dp) : MATLAB Function  TreatAsAtomicUnit=on
  dp_path_s_final : Outport
  dp_path_l_final : Outport  Port=2
  dp_path_dl_final : Outport  Port=3
  dp_path_ddl_final : Outport  Port=4
  wires:
  [plan_start_s] -> path decision with dynamic planning(dp)/3(plan_start_s)
  path decision with dynamic planning(dp)/1(dp_path_s) -> [dp_path_s_init]
  increase DP path nodes/2(dp_path_l_final) -> [dp_path_l_final]
  [static_obs_l_set] -> path decision with dynamic planning(dp)/2(obs_l_set)
  [plan_start_ddl] -> path decision with dynamic planning(dp)/6(plan_start_dll)
  [plan_start_l] -> path decision with dynamic planning(dp)/4(plan_start_l)
  [static_obs_s_set] -> path decision with dynamic planning(dp)/1(obs_s_set)
  [plan_start_dl] -> increase DP path nodes/5(plan_start_dl)
  increase DP path nodes/4(dp_path_ddl_final) -> [dp_path_ddl_final]
  increase DP path nodes/1(dp_path_s_final) -> [dp_path_s_final]
  increase DP path nodes/3(dp_path_dl_final) -> [dp_path_dl_final]
  path decision with dynamic planning(dp)/2(dp_path_l) -> [dp_path_l_init]
  [plan_start_l] -> increase DP path nodes/4(plan_start_l)
  [plan_start_ddl] -> increase DP path nodes/6(plan_start_ddl)
  [plan_start_dl] -> path decision with dynamic planning(dp)/5(plan_start_dl)
  [plan_start_s] -> increase DP path nodes/3(plan_start_s)
  [dp_path_l_init] -> increase DP path nodes/2(dp_path_l_init)
  [dp_path_s_init] -> increase DP path nodes/1(dp_path_s_init)
  static_obs_s_set/1 -> [static_obs_s_set]
  static_obs_l_set/1 -> [static_obs_l_set]
  plan_start_s/1 -> [plan_start_s]
  plan_start_l/1 -> [plan_start_l]
  plan_start_dl/1 -> [plan_start_dl]
  plan_start_ddl/1 -> [plan_start_ddl]
  [dp_path_s_final] -> dp_path_s_final/1
  [dp_path_l_final] -> dp_path_l_final/1
  [dp_path_dl_final] -> dp_path_dl_final/1
  [dp_path_ddl_final] -> dp_path_ddl_final/1
  [dp_cost_collision] -> path decision with dynamic planning(dp)/7(w_cost_collision)
  [dp_cost_dl] -> path decision with dynamic planning(dp)/8(w_cost_smooth_dl)
  [dp_cost_ddl] -> path decision with dynamic planning(dp)/9(w_cost_smooth_ddl)
  [dp_cost_dddl] -> path decision with dynamic planning(dp)/10(w_cost_smooth_dddl)
  [dp_cost_ref] -> path decision with dynamic planning(dp)/11(w_cost_ref)
  [dp_row] -> path decision with dynamic planning(dp)/12(row)
  [dp_col] -> path decision with dynamic planning(dp)/13(col)
  [dp_sample_s] -> path decision with dynamic planning(dp)/14(sample_s)
  [dp_sample_l] -> path decision with dynamic planning(dp)/15(sample_l)
  dp_cost_dl/1 -> [dp_cost_dl]
  dp_cost_ddl/1 -> [dp_cost_ddl]
  dp_cost_dddl/1 -> [dp_cost_dddl]
  dp_cost_ref/1 -> [dp_cost_ref]
  dp_row/1 -> [dp_row]
  dp_col/1 -> [dp_col]
  dp_sample_l/1 -> [dp_sample_l]
  dp_sample_s/1 -> [dp_sample_s]
  dp_cost_collision/1 -> [dp_cost_collision]

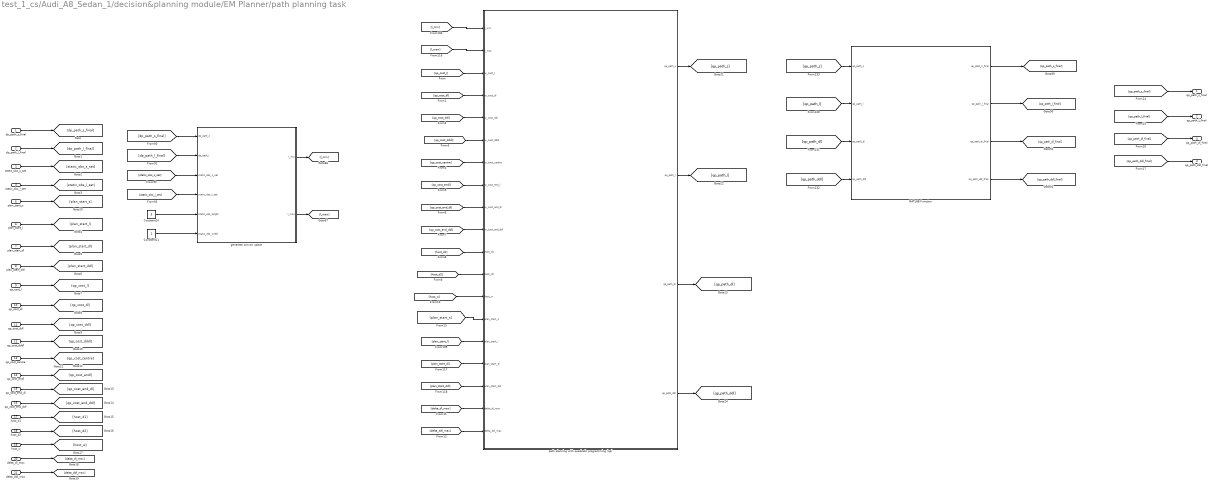
== system test_1_cs/Audi_A8_Sedan_1/decision&planning module/EM Planner/path planning task ==
  dp_path_s_final : Inport
  dp_path_l_final : Inport  Port=2
  static_obs_s_set : Inport  Port=3
  static_obs_l_set : Inport  Port=4
  plan_start_s : Inport  Port=5
  plan_start_l : Inport  Port=6
  plan_start_dl : Inport  Port=7
  plan_start_ddl : Inport  Port=8
  qp_cost_l : Inport  Port=9
  qp_cost_dl : Inport  Port=10
  qp_cost_ddl : Inport  Port=11
  qp_cost_dddl : Inport  Port=12
  qp_cost_centre : Inport  Port=13
  qp_cost_endl : Inport  Port=14
  qp_cost_end_dl : Inport  Port=15
  qp_cost_end_ddl : Inport  Port=16
  host_d1 : Inport  Port=17
  host_d2 : Inport  Port=18
  host_w : Inport  Port=19
  delta_dl_max : Inport  Port=20
  delta_ddl_max : Inport  Port=21
  Constant10 : Constant  Value=5
  Constant11 : Constant  Value=2
  MATLAB Function : MATLAB Function  TreatAsAtomicUnit=on
  generate convex space : MATLAB Function  TreatAsAtomicUnit=on
  path planning with quadratic programming (qp) : MATLAB Function  TreatAsAtomicUnit=on
  qp_path_s_final : Outport
  qp_path_l_final : Outport  Port=2
  qp_path_dl_final : Outport  Port=3
  qp_path_ddl_final : Outport  Port=4
  wires:
  generate convex space/2(l_max) -> [l_max]
  Constant11/1 -> generate convex space/6(static_obs_width)
  Constant10/1 -> generate convex space/5(static_obs_length)
  [static_obs_l_set] -> generate convex space/4(static_obs_l_set)
  [dp_path_s_final] -> generate convex space/1(dp_path_s)
  [plan_start_l] -> path planning with quadratic programming (qp)/15(plan_start_l)
  generate convex space/1(l_min) -> [l_min]
  [static_obs_s_set] -> generate convex space/3(static_obs_s_set)
  [dp_path_l_final] -> generate convex space/2(dp_path_l)
  [plan_start_dl] -> path planning with quadratic programming (qp)/16(plan_start_dl)
  [l_max] -> path planning with quadratic programming (qp)/2(l_max)
  [l_min] -> path planning with quadratic programming (qp)/1(l_min)
  [plan_start_ddl] -> path planning with quadratic programming (qp)/17(plan_start_ddl)
  dp_path_s_final/1 -> [dp_path_s_final]
  dp_path_l_final/1 -> [dp_path_l_final]
  static_obs_s_set/1 -> [static_obs_s_set]
  static_obs_l_set/1 -> [static_obs_l_set]
  plan_start_l/1 -> [plan_start_l]
  plan_start_dl/1 -> [plan_start_dl]
  plan_start_ddl/1 -> [plan_start_ddl]
  [qp_cost_l] -> path planning with quadratic programming (qp)/3(w_cost_l)
  [qp_cost_dl] -> path planning with quadratic programming (qp)/4(w_cost_dl)
  [qp_cost_ddl] -> path planning with quadratic programming (qp)/5(w_cost_ddl)
  [qp_cost_dddl] -> path planning with quadratic programming (qp)/6(w_cost_dddl)
  [qp_cost_centre] -> path planning with quadratic programming (qp)/7(w_cost_centre)
  [qp_cost_endl] -> path planning with quadratic programming (qp)/8(w_cost_end_l)
  [qp_cost_end_dl] -> path planning with quadratic programming (qp)/9(w_cost_end_dl)
  [qp_cost_end_ddl] -> path planning with quadratic programming (qp)/10(w_cost_end_ddl)
  [host_d1] -> path planning with quadratic programming (qp)/11(host_d1)
  [host_d2] -> path planning with quadratic programming (qp)/12(host_d2)
  [host_w] -> path planning with quadratic programming (qp)/13(host_w)
  qp_cost_l/1 -> [qp_cost_l]
  qp_cost_dl/1 -> [qp_cost_dl]
  qp_cost_ddl/1 -> [qp_cost_ddl]
  qp_cost_dddl/1 -> [qp_cost_dddl]
  qp_cost_centre/1 -> [qp_cost_centre]
  qp_cost_endl/1 -> [qp_cost_endl]
  qp_cost_end_dl/1 -> [qp_cost_end_dl]
  qp_cost_end_ddl/1 -> [qp_cost_end_ddl]
  host_d1/1 -> [host_d1]
  host_d2/1 -> [host_d2]
  host_w/1 -> [host_w]
  [delta_dl_max] -> path planning with quadratic programming (qp)/18(delta_dl_max)
  [delta_ddl_max] -> path planning with quadratic programming (qp)/19(delta_ddl_max)
  delta_dl_max/1 -> [delta_dl_max]
  delta_ddl_max/1 -> [delta_ddl_max]
  plan_start_s/1 -> [plan_start_s]
  [plan_start_s] -> path planning with quadratic programming (qp)/14(plan_start_s)
  MATLAB Function/1(qp_path_s_final) -> [qp_path_s_final]
  MATLAB Function/3(qp_path_dl_final) -> [qp_path_dl_final]
  [qp_path_s] -> MATLAB Function/1(qp_path_s)
  [qp_path_ddl] -> MATLAB Function/4(qp_path_ddl)
  MATLAB Function/2(qp_path_l_final) -> [qp_path_l_final]
  [qp_path_dl] -> MATLAB Function/3(qp_path_dl)
  MATLAB Function/4(qp_path_ddl_final) -> [qp_path_ddl_final]
  [qp_path_l] -> MATLAB Function/2(qp_path_l)
  [qp_path_s_final] -> qp_path_s_final/1
  [qp_path_l_final] -> qp_path_l_final/1
  [qp_path_dl_final] -> qp_path_dl_final/1
  [qp_path_ddl_final] -> qp_path_ddl_final/1
  path planning with quadratic programming (qp)/1(qp_path_s) -> [qp_path_s]
  path planning with quadratic programming (qp)/2(qp_path_l) -> [qp_path_l]
  path planning with quadratic programming (qp)/3(qp_path_dl) -> [qp_path_dl]
  path planning with quadratic programming (qp)/4(qp_path_ddl) -> [qp_path_ddl]

== system test_1_cs/Audi_A8_Sedan_3/SELF_Demux/compas converter/cart2compas ==
  Angle [deg] : Inport
  Constant : Constant  Value=90
  Constant1 : Constant  Value=360
  Gain : Gain  Gain=1/360
  Gain1 : Gain  Gain=360
  Gain2 : Gain  Gain=-1
  Rounding Function : Rounding
  Sum : Sum  Inputs=|-+
  Sum1 : Sum  Inputs=-+|
  Sum2 : Sum  Inputs=++|
  heading [deg] : Outport
  wires:
  Gain/1 -> Rounding Function/1
  Rounding Function/1 -> Gain1/1
  Gain1/1 -> Sum/1
  Angle [deg]/1 -> Sum1/2
  Sum/1 -> Gain2/1
  Sum1/1 -> Gain/1, Sum/2
  Constant/1 -> Sum1/1
  Gain2/1 -> Sum2/2
  Constant1/1 -> Sum2/1
  Sum2/1 -> heading [deg]/1

== system test_1_cs/Audi_A8_Sedan_3/Trajectories/Traj2State1/Traj2State2 ==
  traj : Inport
  MuxState : Subsystem
  Traj2MuxState_Ext : Subsystem
  state : Outport
  wires:
  Traj2MuxState_Ext/9(Y [rad]) -> MuxState/9(Y [rad])
  Traj2MuxState_Ext/8(P [rad]) -> MuxState/8(P [rad])
  Traj2MuxState_Ext/7(R [rad]) -> MuxState/7(R [rad])
  Traj2MuxState_Ext/6(dz [m/s]) -> MuxState/6(dz [m/s])
  Traj2MuxState_Ext/5(dy [m/s]) -> MuxState/5(dy [m/s])
  Traj2MuxState_Ext/4(dx [m/s]) -> MuxState/4(dx [m/s])
  Traj2MuxState_Ext/3(z [m]) -> MuxState/3(z [m])
  Traj2MuxState_Ext/2(y [m]) -> MuxState/2(y [m])
  Traj2MuxState_Ext/1(x [m]) -> MuxState/1(x [m])
  MuxState/1(state) -> state/1
  traj/1 -> Traj2MuxState_Ext/1(Traj)

== system test_1_cs/Audi_A8_Sedan_4/SELF_Demux/compas converter/cart2compas ==
  Angle [deg] : Inport
  Constant : Constant  Value=90
  Constant1 : Constant  Value=360
  Gain : Gain  Gain=1/360
  Gain1 : Gain  Gain=360
  Gain2 : Gain  Gain=-1
  Rounding Function : Rounding
  Sum : Sum  Inputs=|-+
  Sum1 : Sum  Inputs=-+|
  Sum2 : Sum  Inputs=++|
  heading [deg] : Outport
  wires:
  Gain/1 -> Rounding Function/1
  Rounding Function/1 -> Gain1/1
  Gain1/1 -> Sum/1
  Angle [deg]/1 -> Sum1/2
  Sum/1 -> Gain2/1
  Sum1/1 -> Gain/1, Sum/2
  Constant/1 -> Sum1/1
  Gain2/1 -> Sum2/2
  Constant1/1 -> Sum2/1
  Sum2/1 -> heading [deg]/1

== system test_1_cs/Audi_A8_Sedan_4/Trajectories/Traj2State1/Traj2State2 ==
  traj : Inport
  MuxState : Subsystem
  Traj2MuxState_Ext : Subsystem
  state : Outport
  wires:
  Traj2MuxState_Ext/9(Y [rad]) -> MuxState/9(Y [rad])
  Traj2MuxState_Ext/8(P [rad]) -> MuxState/8(P [rad])
  Traj2MuxState_Ext/7(R [rad]) -> MuxState/7(R [rad])
  Traj2MuxState_Ext/6(dz [m/s]) -> MuxState/6(dz [m/s])
  Traj2MuxState_Ext/5(dy [m/s]) -> MuxState/5(dy [m/s])
  Traj2MuxState_Ext/4(dx [m/s]) -> MuxState/4(dx [m/s])
  Traj2MuxState_Ext/3(z [m]) -> MuxState/3(z [m])
  Traj2MuxState_Ext/2(y [m]) -> MuxState/2(y [m])
  Traj2MuxState_Ext/1(x [m]) -> MuxState/1(x [m])
  MuxState/1(state) -> state/1
  traj/1 -> Traj2MuxState_Ext/1(Traj)

== system test_1_cs/Box_1/SELF_Demux/compas converter/cart2compas ==
  Angle [deg] : Inport
  Constant : Constant  Value=90
  Constant1 : Constant  Value=360
  Gain : Gain  Gain=1/360
  Gain1 : Gain  Gain=360
  Gain2 : Gain  Gain=-1
  Rounding Function : Rounding
  Sum : Sum  Inputs=|-+
  Sum1 : Sum  Inputs=-+|
  Sum2 : Sum  Inputs=++|
  heading [deg] : Outport
  wires:
  Gain/1 -> Rounding Function/1
  Rounding Function/1 -> Gain1/1
  Gain1/1 -> Sum/1
  Angle [deg]/1 -> Sum1/2
  Sum/1 -> Gain2/1
  Sum1/1 -> Gain/1, Sum/2
  Constant/1 -> Sum1/1
  Gain2/1 -> Sum2/2
  Constant1/1 -> Sum2/1
  Sum2/1 -> heading [deg]/1

== system test_1_cs/Box_2/SELF_Demux/compas converter/cart2compas ==
  Angle [deg] : Inport
  Constant : Constant  Value=90
  Constant1 : Constant  Value=360
  Gain : Gain  Gain=1/360
  Gain1 : Gain  Gain=360
  Gain2 : Gain  Gain=-1
  Rounding Function : Rounding
  Sum : Sum  Inputs=|-+
  Sum1 : Sum  Inputs=-+|
  Sum2 : Sum  Inputs=++|
  heading [deg] : Outport
  wires:
  Gain/1 -> Rounding Function/1
  Rounding Function/1 -> Gain1/1
  Gain1/1 -> Sum/1
  Angle [deg]/1 -> Sum1/2
  Sum/1 -> Gain2/1
  Sum1/1 -> Gain/1, Sum/2
  Constant/1 -> Sum1/1
  Gain2/1 -> Sum2/2
  Constant1/1 -> Sum2/1
  Sum2/1 -> heading [deg]/1

== system test_1_cs/Box_3/SELF_Demux/compas converter/cart2compas ==
  Angle [deg] : Inport
  Constant : Constant  Value=90
  Constant1 : Constant  Value=360
  Gain : Gain  Gain=1/360
  Gain1 : Gain  Gain=360
  Gain2 : Gain  Gain=-1
  Rounding Function : Rounding
  Sum : Sum  Inputs=|-+
  Sum1 : Sum  Inputs=-+|
  Sum2 : Sum  Inputs=++|
  heading [deg] : Outport
  wires:
  Gain/1 -> Rounding Function/1
  Rounding Function/1 -> Gain1/1
  Gain1/1 -> Sum/1
  Angle [deg]/1 -> Sum1/2
  Sum/1 -> Gain2/1
  Sum1/1 -> Gain/1, Sum/2
  Constant/1 -> Sum1/1
  Gain2/1 -> Sum2/2
  Constant1/1 -> Sum2/1
  Sum2/1 -> heading [deg]/1

== system test_1_cs/Box_4/SELF_Demux/compas converter/cart2compas ==
  Angle [deg] : Inport
  Constant : Constant  Value=90
  Constant1 : Constant  Value=360
  Gain : Gain  Gain=1/360
  Gain1 : Gain  Gain=360
  Gain2 : Gain  Gain=-1
  Rounding Function : Rounding
  Sum : Sum  Inputs=|-+
  Sum1 : Sum  Inputs=-+|
  Sum2 : Sum  Inputs=++|
  heading [deg] : Outport
  wires:
  Gain/1 -> Rounding Function/1
  Rounding Function/1 -> Gain1/1
  Gain1/1 -> Sum/1
  Angle [deg]/1 -> Sum1/2
  Sum/1 -> Gain2/1
  Sum1/1 -> Gain/1, Sum/2
  Constant/1 -> Sum1/1
  Gain2/1 -> Sum2/2
  Constant1/1 -> Sum2/1
  Sum2/1 -> heading [deg]/1

== system test_1_cs/Box_5/SELF_Demux/compas converter/cart2compas ==
  Angle [deg] : Inport
  Constant : Constant  Value=90
  Constant1 : Constant  Value=360
  Gain : Gain  Gain=1/360
  Gain1 : Gain  Gain=360
  Gain2 : Gain  Gain=-1
  Rounding Function : Rounding
  Sum : Sum  Inputs=|-+
  Sum1 : Sum  Inputs=-+|
  Sum2 : Sum  Inputs=++|
  heading [deg] : Outport
  wires:
  Gain/1 -> Rounding Function/1
  Rounding Function/1 -> Gain1/1
  Gain1/1 -> Sum/1
  Angle [deg]/1 -> Sum1/2
  Sum/1 -> Gain2/1
  Sum1/1 -> Gain/1, Sum/2
  Constant/1 -> Sum1/1
  Gain2/1 -> Sum2/2
  Constant1/1 -> Sum2/1
  Sum2/1 -> heading [deg]/1

== system test_1_cs/Box_6/SELF_Demux/compas converter/cart2compas ==
  Angle [deg] : Inport
  Constant : Constant  Value=90
  Constant1 : Constant  Value=360
  Gain : Gain  Gain=1/360
  Gain1 : Gain  Gain=360
  Gain2 : Gain  Gain=-1
  Rounding Function : Rounding
  Sum : Sum  Inputs=|-+
  Sum1 : Sum  Inputs=-+|
  Sum2 : Sum  Inputs=++|
  heading [deg] : Outport
  wires:
  Gain/1 -> Rounding Function/1
  Rounding Function/1 -> Gain1/1
  Gain1/1 -> Sum/1
  Angle [deg]/1 -> Sum1/2
  Sum/1 -> Gain2/1
  Sum1/1 -> Gain/1, Sum/2
  Constant/1 -> Sum1/1
  Gain2/1 -> Sum2/2
  Constant1/1 -> Sum2/1
  Sum2/1 -> heading [deg]/1

== system test_1_cs/Box_7/SELF_Demux/compas converter/cart2compas ==
  Angle [deg] : Inport
  Constant : Constant  Value=90
  Constant1 : Constant  Value=360
  Gain : Gain  Gain=1/360
  Gain1 : Gain  Gain=360
  Gain2 : Gain  Gain=-1
  Rounding Function : Rounding
  Sum : Sum  Inputs=|-+
  Sum1 : Sum  Inputs=-+|
  Sum2 : Sum  Inputs=++|
  heading [deg] : Outport
  wires:
  Gain/1 -> Rounding Function/1
  Rounding Function/1 -> Gain1/1
  Gain1/1 -> Sum/1
  Angle [deg]/1 -> Sum1/2
  Sum/1 -> Gain2/1
  Sum1/1 -> Gain/1, Sum/2
  Constant/1 -> Sum1/1
  Gain2/1 -> Sum2/2
  Constant1/1 -> Sum2/1
  Sum2/1 -> heading [deg]/1

== system test_1_cs/Child_Regular_Leaning_1/SELF_Demux/compas converter/cart2compas ==
  Angle [deg] : Inport
  Constant : Constant  Value=90
  Constant1 : Constant  Value=360
  Gain : Gain  Gain=1/360
  Gain1 : Gain  Gain=360
  Gain2 : Gain  Gain=-1
  Rounding Function : Rounding
  Sum : Sum  Inputs=|-+
  Sum1 : Sum  Inputs=-+|
  Sum2 : Sum  Inputs=++|
  heading [deg] : Outport
  wires:
  Gain/1 -> Rounding Function/1
  Rounding Function/1 -> Gain1/1
  Gain1/1 -> Sum/1
  Angle [deg]/1 -> Sum1/2
  Sum/1 -> Gain2/1
  Sum1/1 -> Gain/1, Sum/2
  Constant/1 -> Sum1/1
  Gain2/1 -> Sum2/2
  Constant1/1 -> Sum2/1
  Sum2/1 -> heading [deg]/1

== system test_1_cs/Child_Regular_Leaning_1/Trajectories/Traj2State1/Traj2State2 ==
  traj : Inport
  MuxState : Subsystem
  Traj2MuxState_Ext : Subsystem
  state : Outport
  wires:
  Traj2MuxState_Ext/9(Y [rad]) -> MuxState/9(Y [rad])
  Traj2MuxState_Ext/8(P [rad]) -> MuxState/8(P [rad])
  Traj2MuxState_Ext/7(R [rad]) -> MuxState/7(R [rad])
  Traj2MuxState_Ext/6(dz [m/s]) -> MuxState/6(dz [m/s])
  Traj2MuxState_Ext/5(dy [m/s]) -> MuxState/5(dy [m/s])
  Traj2MuxState_Ext/4(dx [m/s]) -> MuxState/4(dx [m/s])
  Traj2MuxState_Ext/3(z [m]) -> MuxState/3(z [m])
  Traj2MuxState_Ext/2(y [m]) -> MuxState/2(y [m])
  Traj2MuxState_Ext/1(x [m]) -> MuxState/1(x [m])
  MuxState/1(state) -> state/1
  traj/1 -> Traj2MuxState_Ext/1(Traj)

== system test_1_cs/Female_OverweightAni_1/SELF_Demux/compas converter/cart2compas ==
  Angle [deg] : Inport
  Constant : Constant  Value=90
  Constant1 : Constant  Value=360
  Gain : Gain  Gain=1/360
  Gain1 : Gain  Gain=360
  Gain2 : Gain  Gain=-1
  Rounding Function : Rounding
  Sum : Sum  Inputs=|-+
  Sum1 : Sum  Inputs=-+|
  Sum2 : Sum  Inputs=++|
  heading [deg] : Outport
  wires:
  Gain/1 -> Rounding Function/1
  Rounding Function/1 -> Gain1/1
  Gain1/1 -> Sum/1
  Angle [deg]/1 -> Sum1/2
  Sum/1 -> Gain2/1
  Sum1/1 -> Gain/1, Sum/2
  Constant/1 -> Sum1/1
  Gain2/1 -> Sum2/2
  Constant1/1 -> Sum2/1
  Sum2/1 -> heading [deg]/1

== system test_1_cs/Male_Female_HandInHand_1/SELF_Demux/compas converter/cart2compas ==
  Angle [deg] : Inport
  Constant : Constant  Value=90
  Constant1 : Constant  Value=360
  Gain : Gain  Gain=1/360
  Gain1 : Gain  Gain=360
  Gain2 : Gain  Gain=-1
  Rounding Function : Rounding
  Sum : Sum  Inputs=|-+
  Sum1 : Sum  Inputs=-+|
  Sum2 : Sum  Inputs=++|
  heading [deg] : Outport
  wires:
  Gain/1 -> Rounding Function/1
  Rounding Function/1 -> Gain1/1
  Gain1/1 -> Sum/1
  Angle [deg]/1 -> Sum1/2
  Sum/1 -> Gain2/1
  Sum1/1 -> Gain/1, Sum/2
  Constant/1 -> Sum1/1
  Gain2/1 -> Sum2/2
  Constant1/1 -> Sum2/1
  Sum2/1 -> heading [deg]/1

== system test_1_cs/Male_Female_HandInHand_1/Trajectories/Traj2State1/Traj2State2 ==
  traj : Inport
  MuxState : Subsystem
  Traj2MuxState_Ext : Subsystem
  state : Outport
  wires:
  Traj2MuxState_Ext/9(Y [rad]) -> MuxState/9(Y [rad])
  Traj2MuxState_Ext/8(P [rad]) -> MuxState/8(P [rad])
  Traj2MuxState_Ext/7(R [rad]) -> MuxState/7(R [rad])
  Traj2MuxState_Ext/6(dz [m/s]) -> MuxState/6(dz [m/s])
  Traj2MuxState_Ext/5(dy [m/s]) -> MuxState/5(dy [m/s])
  Traj2MuxState_Ext/4(dx [m/s]) -> MuxState/4(dx [m/s])
  Traj2MuxState_Ext/3(z [m]) -> MuxState/3(z [m])
  Traj2MuxState_Ext/2(y [m]) -> MuxState/2(y [m])
  Traj2MuxState_Ext/1(x [m]) -> MuxState/1(x [m])
  MuxState/1(state) -> state/1
  traj/1 -> Traj2MuxState_Ext/1(Traj)
